simulink model "Task2"  (R2021a)
settings: Solver=VariableStepAuto  StartTime=0.0  StopTime=10.0  RelTol=1e-3
settings Model: Creator=Alaa  LastModifiedBy=Alaa

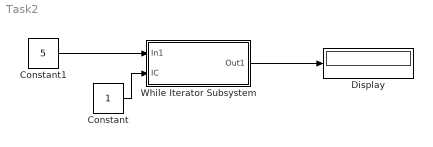
== system Task2 ==
  Constant : Constant
  Constant1 : Constant  Value=5
  Display : Display
  While Iterator Subsystem : Subsystem  TreatAsAtomicUnit=on
  wires:
  Constant/1 -> While Iterator Subsystem/2(IC)
  Constant1/1 -> While Iterator Subsystem/1(In1)
  While Iterator Subsystem/1(Out1) -> Display/1

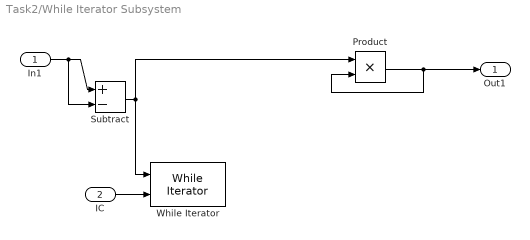
== system Task2/While Iterator Subsystem ==
  In1 : Inport
  IC : Inport  Port=2
  Product : Product
  Subtract : Sum  Inputs=+-
  While Iterator : WhileIterator  MaxIters=10
  Out1 : Outport
  wires:
  IC/1 -> While Iterator/2
  Product/1 -> Product/2, Out1/1
  In1/1 -> Subtract/2, Subtract/1
  Subtract/1 -> While Iterator/1, Product/1
